simulink model "q7"  (R2019a)
settings: Solver=VariableStepAuto  StartTime=0.0  StopTime=0.01  RelTol=1e-3
settings Model: Creator=ADMIN  LastModifiedBy=ADMIN

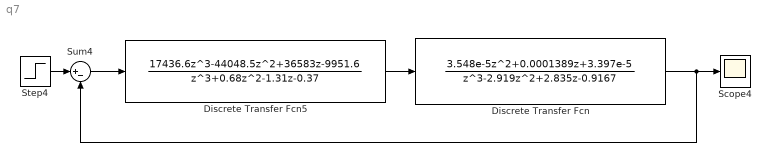
== system q7 ==
  Discrete Transfer Fcn : DiscreteTransferFcn  Numerator=[3.548e-5 0.0001389 3.397e-5]  Denominator=[1 -2.919 2.835 -0.9167]  SampleTime=0.001
  Discrete Transfer Fcn5 : DiscreteTransferFcn  Numerator=[17436.6 -44048.5 36583 -9951.6]  Denominator=[1 0.68 -1.31 -0.37]  SampleTime=0.001
  Scope4 : Scope
  Step4 : Step  Time=0  SampleTime=0.001
  Sum4 : Sum  Inputs=|+-
  wires:
  Discrete Transfer Fcn/1 -> Scope4/1, Sum4/2
  Step4/1 -> Sum4/1
  Sum4/1 -> Discrete Transfer Fcn5/1
  Discrete Transfer Fcn5/1 -> Discrete Transfer Fcn/1
